simulink model "Simple_Model_Packaging_4_1"  (R2022b)
settings: Solver=VariableStepAuto  StartTime=0.0  StopTime=0.03  RelTol=1e-3
InitFcn:
  | Parameter_Initialize_4
undefined symbols (not defined in the file or in its folder): gcbh, model, rcfiltgaincompat, rsgenpoly
libraries: dspobslib x11, commdigbbndpm3 x6, commdigbbndam3 x6, simulink x5, commblkintrlv2 x4, commfilt2 x4, commsynccomp2 x3, commblkcod2 x2, commrandsrc3 x2, commseqgen3 x2, commchan3 x1, dspsigops x1
(part 1 of 2)
settings Model: Creator=89778  LastModifiedBy=z0y

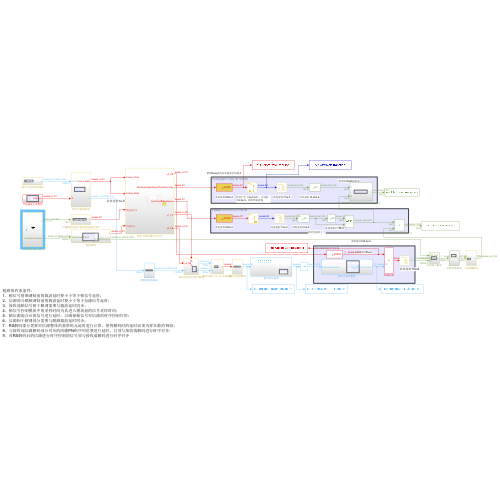
[thumbnail: Simulink's stored preview of the top-level diagram]
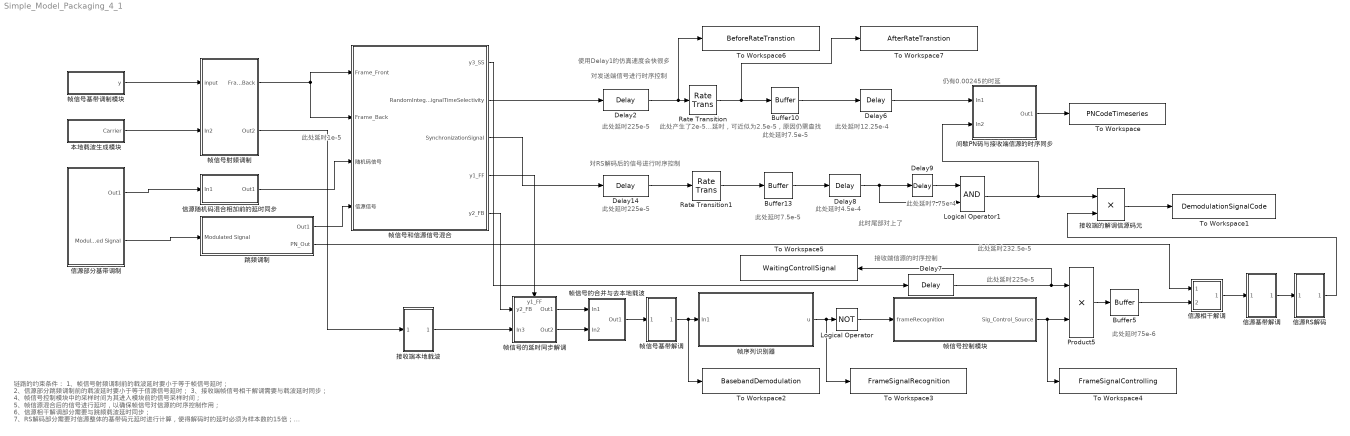
== system Simple_Model_Packaging_4_1 ==
  note: 此时尾部对上了
  note: 此处产生了2e-5延时，可近似为2.5e-5，原因仍需查找
  note: 仍有0.00245的时延
  note: 使用Delay1的仿真速度会快很多
  note: 对发送端信号进行时序控制
  note: 链路的约束条件：
      | 1、帧信号射频调制前的载波延时要小于等于帧信号延时；
      | 2、信源部分跳频调制前的载波延时要小于等于信源信号延时；
      | 3、接收端帧信号相干解调需要与载波延时同步；
      | 4、帧信号控制模块中的采样时间为其进入模块前的信号采样时间；
      | 5、帧信源混合后的信号进行延时，以确保帧信号对信源的时序控制作用；
      | 6、信源相干解调部分需要与跳频载波延时同步；
      | 7、RS解码部分需要对信源整体的基带码元延时进行计算，使得解码时的延时必须为样本数的15倍；
      | 8、与接收端信源解码部分对应的间歇PN码序列也要进行延时，且须与接收端解码进行时序对齐；
      | 9、对RS解码后的信源进行时序控制的信号须与接收端解码进行时序对齐
  note: 此处延时75e-6
  note: 此处延时1e-5
  note: 对RS解码后的信号进行时序控制
  note: 接收端信源的时序控制
  note: 此处延时225e-5
  note: 此处延时225e-5
  note: 此处延时7.5e-5
  note: 此处延时7.5e-5
  note: 此处延时7.75e-4
  note: 此处延时232.5e-5
  note: 此处延时225e-5
  note: 此处延时12.25e-4
  note: 此处延时4.5e-4
  Buffer10 : Buffer  N=model.parameter.Buffer10.Output_buffer_size  OutputFrames=off
  Buffer13 : Buffer  N=model.parameter.Buffer13.Output_buffer_size  OutputFrames=off
  Buffer5 : Buffer  N=model.parameter.Beffer5.Output_buffer_size  OutputFrames=off
  Delay14 : dspobslib/Delay  InputProcessing=Columns as channels (frame based)  dly_unit=Samples  delay=model.parameter.Delay14.Output_buffer_size  ic_detail=off  dif_ic_for_ch=on  dif_ic_for_dly=off  ic=0  reset_popup=None
  Delay2 : dspobslib/Delay  InputProcessing=Columns as channels (frame based)  dly_unit=Samples  delay=model.parameter.Delay2.Output_buffer_size  ic_detail=off  dif_ic_for_ch=on  dif_ic_for_dly=off  ic=0  reset_popup=None
  Delay6 : dspobslib/Delay  InputProcessing=Columns as channels (frame based)  dly_unit=Samples  delay=model.parameter.Delay6.Output_buffer_size  ic_detail=off  dif_ic_for_ch=on  dif_ic_for_dly=off  ic=0  reset_popup=None
  Delay7 : dspobslib/Delay  InputProcessing=Columns as channels (frame based)  dly_unit=Samples  delay=model.parameter.Delay7.samples_length  ic_detail=off  dif_ic_for_ch=on  dif_ic_for_dly=off  ic=0  reset_popup=None
  Delay8 : dspobslib/Delay  InputProcessing=Columns as channels (frame based)  dly_unit=Samples  delay=model.parameter.Delay8.Output_buffer_size  ic_detail=off  dif_ic_for_ch=on  dif_ic_for_dly=off  ic=0  reset_popup=None
  Delay9 : dspobslib/Delay  InputProcessing=Columns as channels (frame based)  dly_unit=Samples  delay=model.parameter.Delay9.Output_buffer_size  ic_detail=off  dif_ic_for_ch=on  dif_ic_for_dly=off  ic=0  reset_popup=None
  Logical Operator : Logic  Operator=NOT  AllPortsSameDT=off  OutDataTypeStr=boolean
  Logical Operator1 : Logic  AllPortsSameDT=off  OutDataTypeStr=boolean
  Product5 : Product
  Rate Transition : RateTransition  OutPortSampleTime=model.parameter.Rate_Transition.Ts
  Rate Transition1 : RateTransition  OutPortSampleTime=model.parameter.Rate_Transition1.Ts
  To Workspace : ToWorkspace  VariableName=PNCodeTimeseries  SaveFormat=Timeseries  SampleTime=-1
  To Workspace1 : ToWorkspace  VariableName=DemodulationSignalCode  SaveFormat=Timeseries  SampleTime=-1
  To Workspace2 : ToWorkspace  VariableName=BasebandDemodulation  SaveFormat=Timeseries  SampleTime=-1
  To Workspace3 : ToWorkspace  VariableName=FrameSignalRecognition  SaveFormat=Timeseries  SampleTime=-1
  To Workspace4 : ToWorkspace  VariableName=FrameSignalControlling  SaveFormat=Timeseries  SampleTime=-1
  To Workspace5 : ToWorkspace  VariableName=WaitingControllSignal  SaveFormat=Timeseries  SampleTime=-1
  To Workspace6 : ToWorkspace  VariableName=BeforeRateTranstion  SaveFormat=Timeseries  SampleTime=-1
  To Workspace7 : ToWorkspace  VariableName=AfterRateTranstion  SaveFormat=Timeseries  SampleTime=-1
  信源RS解码 : Subsystem
  信源基带解调 : Subsystem
  信源相干解调 : Subsystem
  信源部分基带调制 : Subsystem
  信源随机码混合相加前的延时同步 : Subsystem
  帧信号和信源信号混合 : Subsystem
  帧信号基带解调 : Subsystem
  帧信号基带调制模块 : Subsystem
  帧信号射频调制 : Subsystem
  帧信号控制模块 : Subsystem
  帧信号的合并与去本地载波 : Subsystem
  帧信号的延时同步解调 : Subsystem
      settings: PortSchema="{\"entries\":[{\"content\":{\"sides\":[{\"content\":{\"connectorIds\":[\"In1\",\"In2\"]},\"type\":\"ConnectorPlacement.EquallySpacedRectSide\",\"uuid\":\"7f942f1a-e4af-4868-9b8e-272828cafa58\"},{\"content\":{\"connectorIds\":[\"Out1\",\"Out2\"],\"side\":\"RIGHT\"},\"type\":\"ConnectorPlacement.EquallySpacedRectSide\",\"uuid\":\"5681018a-c54d-4fc6-9bb9-b0c232ec8fca\"},{\"content\":{\"connectorIds\":[\"In3\"],\"side\":\"TOP\"},\"type\":\"ConnectorPlacement.EquallySpacedRectSide\",\"uuid\":\"54722782-433f-4e80-acce-11fefe357297\"}]},\"type\":\"ConnectorPlacement.EquallySpacedConnector\",\"uuid\":\"571cebd7-6074-490f-8ff4-11297431766f\"}],\"packageUris\":[\"http://schema.mathworks.com/mf0/Connector/R2020b\"],\"version\":\"1.0\"}"
  帧序列识别器 : Subsystem
  接收端本地载波 : Subsystem
  接收端的解调信源码元 : Product
  本地载波生成模块 : Subsystem
  跳频调制 : Subsystem
  间歇PN码与接收端信源的时序同步 : Subsystem
  wires:
  Product5/1 -> Buffer5/1
  帧信号和信源信号混合/1(y3_SS) -> Delay7/1
  帧序列识别器/1(u) -> To Workspace3/1, Logical Operator/1
  Delay7/1 -> To Workspace5/1, Product5/1
  Buffer13/1 -> Delay8/1
  帧信号基带调制模块/1(y) -> 帧信号射频调制/1(input)
  本地载波生成模块/1(Carrier) -> 帧信号射频调制/2(In2)
  跳频调制/1(Out1) -> 帧信号和信源信号混合/4(信源信号)
  帧信号射频调制/2(Out2) -> 接收端本地载波/1(In1)
  信源部分基带调制/1(Out1) -> 信源随机码混合相加前的延时同步/1(In1)
  信源随机码混合相加前的延时同步/1(Out1) -> 帧信号和信源信号混合/3(随机码信号)
  接收端本地载波/1(Out1) -> 帧信号的延时同步解调/2(In3)
  帧信号的延时同步解调/1(Out1) -> 帧信号的合并与去本地载波/1(In1)
  帧信号的延时同步解调/2(Out2) -> 帧信号的合并与去本地载波/2(In2)
  帧信号的合并与去本地载波/1(Out1) -> 帧信号基带解调/1(In1)
  帧信号基带解调/1(Out1) -> To Workspace2/1, 帧序列识别器/1(In1)
  Logical Operator/1 -> 帧信号控制模块/1(frameRecognition)
  帧信号控制模块/1(Sig_Control_Source) -> To Workspace4/1, Product5/2
  信源RS解码/1(Out1) -> 接收端的解调信源码元/2
  Buffer5/1 -> 信源相干解调/2(In2)
  信源相干解调/1(Out1) -> 信源基带解调/1(In1)
  帧信号和信源信号混合/4(y1_FF) -> 帧信号的延时同步解调/3(y1_FF)
  帧信号和信源信号混合/5(y2_FB) -> 帧信号的延时同步解调/1(y2_FB)
  跳频调制/2(PN_Out) -> 信源相干解调/1(PN_Out)
  Delay14/1 -> Rate Transition1/1
  帧信号和信源信号混合/2(RandomIntegerSignalTimeSelectivity) -> Delay2/1
  Rate Transition/1 -> To Workspace7/1, Buffer10/1
  Delay2/1 -> To Workspace6/1, Rate Transition/1
  Rate Transition1/1 -> Buffer13/1
  帧信号和信源信号混合/3(SynchronizationSignal) -> Delay14/1
  信源基带解调/1(Out1) -> 信源RS解码/1(In1)
  Buffer10/1 -> Delay6/1
  Delay6/1 -> 间歇PN码与接收端信源的时序同步/1(In1)
  Delay9/1 -> Logical Operator1/1
  Delay8/1 -> Logical Operator1/2, Delay9/1
  信源部分基带调制/2(Modulated Signal) -> 跳频调制/1(Modulated Signal)
  帧信号射频调制/1(Frame_Back) -> 帧信号和信源信号混合/2(Frame_Back), 帧信号和信源信号混合/1(Frame_Front)
  Logical Operator1/1 -> 间歇PN码与接收端信源的时序同步/2(In2), 接收端的解调信源码元/1
  间歇PN码与接收端信源的时序同步/1(Out1) -> To Workspace/1
  接收端的解调信源码元/1 -> To Workspace1/1

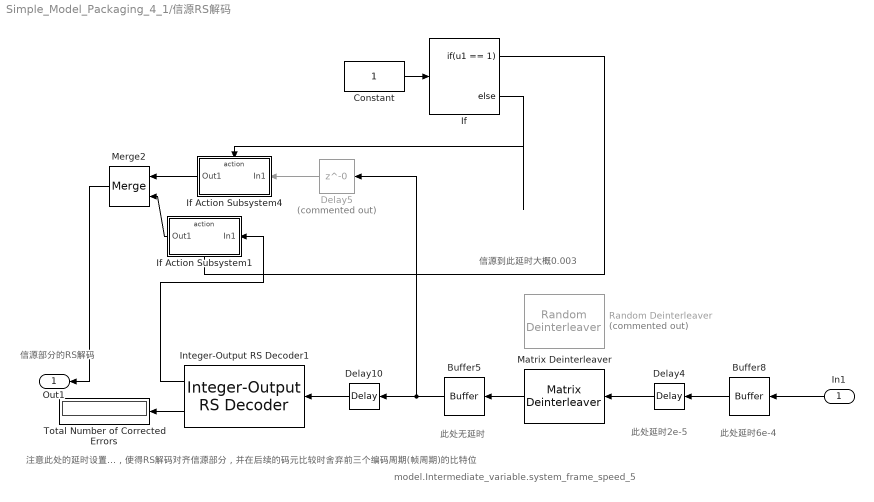
== system Simple_Model_Packaging_4_1/信源RS解码 ==
  note: 信源到此延时大概0.003
  note: model.Intermediate_variable.system_frame_speed_5
  note: 信源部分的RS解码
  note: 注意此处的延时设置，使得RS解码对齐信源部分，并在后续的码元比较时舍弃前三个编码周期(帧周期)的比特位
  note: 此处延时2e-5
  note: 此处无延时
  note: 此处延时6e-4
  In1 : Inport
  Buffer5 : Buffer  N=model.parameter.Buffer5.Output_buffer_size  OutputFrames=off
  Buffer8 : Buffer  N=model.parameter.Buffer8.Output_buffer_size  OutputFrames=off
  Constant : Constant
  Delay10 : dspobslib/Delay  InputProcessing=Columns as channels (frame based)  dly_unit=Samples  delay=model.parameter.Delay10.samples_length  ic_detail=off  dif_ic_for_ch=on  dif_ic_for_dly=off  ic=0  reset_popup=None
  Delay4 : dspobslib/Delay  InputProcessing=Columns as channels (frame based)  dly_unit=Samples  delay=model.parameter.Delay4.samples_length  ic_detail=off  dif_ic_for_ch=on  dif_ic_for_dly=off  ic=0  reset_popup=None
  Delay5 : Delay  Commented=on  DelayLength=0  InitialCondition=0  InputProcessing=Columns as channels (frame based)
  If : If  IfExpression=u1 == 1
  If Action Subsystem1 : Subsystem  TreatAsAtomicUnit=on
  If Action Subsystem4 : Subsystem  TreatAsAtomicUnit=on
  Integer-Output RS Decoder1 : commblkcod2/Integer-Output RS Decoder  n=model.parameter.Integer_Output_RS_Decoder1.Codeword_length  k=model.parameter.Integer_Output_RS_Decoder1.Message_length  specShortening=off  shortenedK=3  specGenPoly=off  genPoly=rsgenpoly(7, 3, [], [], 'double')  specPrimPoly=off  prPoly='X^3 + X + 1'  specPuncture=off  punctVec=[ones(2,1); zeros(2,1)]  specErasurePort=off  showNumErr=on
  Matrix Deinterleaver : commblkintrlv2/Matrix Deinterleaver  StatePerturbationForJacobian=1.0e-05  Nrows=model.parameter.Matrix_Deinterleaver.row_nums  Ncols=model.parameter.Matrix_Deinterleaver.col_nums
  Merge2 : Merge
  Random Deinterleaver : commblkintrlv2/Random Deinterleaver  Commented=on  StatePerturbationForJacobian=1.0e-05  N=120  seed=12345
  Total Number of Corrected Errors : Display
  Out1 : Outport
  wires:
  Integer-Output RS Decoder1/2 -> Total Number of Corrected Errors/1
  Matrix Deinterleaver/1 -> Buffer5/1
  In1/1 -> Buffer8/1
  Buffer8/1 -> Delay4/1
  Delay4/1 -> Matrix Deinterleaver/1
  Delay10/1 -> Integer-Output RS Decoder1/1
  If Action Subsystem4/1(Out1) -> Merge2/1
  Integer-Output RS Decoder1/1 -> If Action Subsystem1/1(In1)
  Buffer5/1 -> Delay5/1, Delay10/1
  Merge2/1 -> Out1/1
  Delay5/1 -> If Action Subsystem4/1(In1)
  If Action Subsystem1/1(Out1) -> Merge2/2
  If/1 -> If Action Subsystem1/Action
  Constant/1 -> If/1
  If/2 -> If Action Subsystem4/Action

== system Simple_Model_Packaging_4_1/信源基带解调 ==
  note: 接收端信源的基带解调
  note: 此处延时2.5e-5
  In1 : Inport
  Baseband Signal Selector Rx : Subsystem
  Merge : Merge  Inputs=3
  OQPSK Demodulator Baseband : commdigbbndpm3/OQPSK Demodulator Baseband  Commented=on  OutType=Integer  Ph=0  Mapping=Gray  pulseShape=Half sine  num=[0.7071, 0.7071]  rolloff=0.2  filterSpan=10  sps=2  RateOptions=Enforce single-rate processing  outDtype2=double
  QPSK Demodulator Baseband : commdigbbndpm3/QPSK Demodulator Baseband  Commented=on  OutType=Integer  DecType=Hard decision  VarSource=Dialog  Variance=1  Dec=Gray  Ph=pi/4  outDtype1=Inherit via internal rule  outDtype2=Inherit via internal rule  derotateFactorWordLen=16  derotateFactorDataTypeStr=Inherit: Same word length as input  derotateFactorLastDataTypeStr=Inherit: Same word length as input
  Raised Cosine Receive Filter1 : commfilt2/Raised Cosine Receive Filter  filtType=Square root  R=model.parameter.Raised_Cosine_Receive_Filter1.Rolloff_factor  filtSpan=model.parameter.Raised_Cosine_Receive_Filter1.Filter_span_in_symbols  N=model.parameter.Raised_Cosine_Receive_Filter1.Input_samples_per_symbol  downFactor=model.parameter.Raised_Cosine_Receive_Filter1.Decimation_fatocr  downOffset=0  filterGain=rcfiltgaincompat(gcbh)  InputProcessing=Columns as channels (frame based)  RateOptions=Enforce single-rate processing  framing=Mute  checkCoeff=off  variableName=rcRxFilt1  currentFiltSpan=10  D=5  inputOffset=0  sampMode=Mute  saveAsFlag=0  rateMode=Downsampling  checkGain=Normalized  launchFVT=on  roundingMode=Floor  overflowMode=off  coeffDataTypeStr=Inherit: Same word length as input  coeffMin=[]  coeffMax=[]  coeffLastDataTypeStr=Inherit: Same word length as input  accumDataTypeStr=Inherit: Same as product output  accumLastDataTypeStr=Inherit: Same as product output  outputDataTypeStr=Inherit: Same as accumulator  outputMin=[]  outputMax=[]  outputLastDataTypeStr=Inherit: Same as accumulator
  Out1 : Outport
  wires:
  Merge/1 -> Out1/1
  In1/1 -> Raised Cosine Receive Filter1/1
  Raised Cosine Receive Filter1/1 -> OQPSK Demodulator Baseband/1, QPSK Demodulator Baseband/1, Baseband Signal Selector Rx/1(In1)
  OQPSK Demodulator Baseband/1 -> Merge/3
  Baseband Signal Selector Rx/1(Out1) -> Merge/1
  QPSK Demodulator Baseband/1 -> Merge/2

== system Simple_Model_Packaging_4_1/信源相干解调 ==
  note: 接收端信源的相干解调
  PN_Out : Inport
  In2 : Inport  Port=2
  Conj1 : Math  Operator=conj
  Delay3 : dspobslib/Delay  InputProcessing=Columns as channels (frame based)  dly_unit=Samples  delay=model.parameter.Delay3.samples_length  ic_detail=off  dif_ic_for_ch=on  dif_ic_for_dly=off  ic=0  reset_popup=None
  Product3 : Product
  Out1 : Outport
  wires:
  PN_Out/1 -> Delay3/1
  Conj1/1 -> Product3/1
  In2/1 -> Product3/2
  Product3/1 -> Out1/1
  Delay3/1 -> Conj1/1

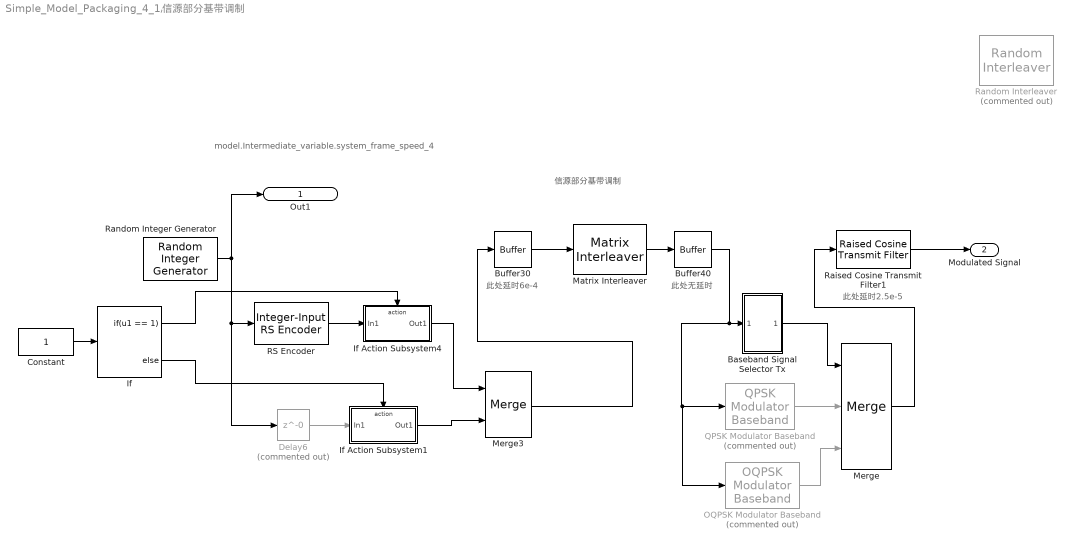
== system Simple_Model_Packaging_4_1/信源部分基带调制 ==
  note: model.Intermediate_variable.system_frame_speed_4
  note: 信源部分基带调制
  note: 此处延时2.5e-5
  note: 此处延时6e-4
  note: 此处无延时
  Baseband Signal Selector Tx : Subsystem
  Buffer30 : Buffer  N=model.parameter.Buffer30.Output_buffer_size  OutputFrames=off
  Buffer40 : Buffer  N=model.parameter.Buffer40.Output_buffer_size  OutputFrames=off
  Constant : Constant
  Delay6 : Delay  Commented=on  DelayLength=0  InitialCondition=0
  If : If  IfExpression=u1 == 1
  If Action Subsystem1 : Subsystem  TreatAsAtomicUnit=on
  If Action Subsystem4 : Subsystem  TreatAsAtomicUnit=on
  Matrix Interleaver : commblkintrlv2/Matrix Interleaver  StatePerturbationForJacobian=1.0e-05  Nrows=model.parameter.Matrix_Interleaver.row_nums  Ncols=model.parameter.Matrix_Interleaver.col_nums
  Merge : Merge  Inputs=3
  Merge3 : Merge
  OQPSK Modulator Baseband : commdigbbndpm3/OQPSK Modulator Baseband  Commented=on  InType=Integer  Ph=0  Mapping=Gray  pulseShape=Half sine  num=[0.7071, 0.7071]  rolloff=0.2  filterSpan=10  sps=2  RateOptions=Enforce single-rate processing  outDtype=double
  QPSK Modulator Baseband : commdigbbndpm3/QPSK Modulator Baseband  Commented=on  InType=Integer  Enc=Gray  Ph=pi/4  outDtype=double  outWordLen=16  outUDDataType=sfix(16)  outFracLenMode=Best precision  outFracLen=15  outDataTypeStr=double  outLastDataTypeStr=double
  RS Encoder : commblkcod2/Integer-Input RS Encoder  n=model.parameter.RS_Encoder.Codeword_length  k=model.parameter.RS_Encoder.Message_length  specShortening=off  shortenedK=3  specGenPoly=off  genPoly=rsgenpoly(7,3)  specPrimPoly=off  prPoly=[1 0 1 1]  specPuncture=off  punctVec=[ones(2,1); zeros(2,1)]
  Raised Cosine Transmit Filter1 : commfilt2/Raised Cosine Transmit Filter  filtType=Square root  R=model.parameter.Raised_Cosine_Transmit_Filter1.Rolloff_factor  filtSpan=model.parameter.Raised_Cosine_Transmit_Filter1.Filter_span_in_symbols  N=model.parameter.Raised_Cosine_Transmit_Filter1.Input_samples_per_symbol  filterGain=rcfiltgaincompat(gcbh)  InputProcessing=Columns as channels (frame based)  RateOptions=Enforce single-rate processing  framing=Mute  checkCoeff=off  variableName=rcTxFilt1  checkGain=Normalized  sampMode=Mute  saveAsFlag=0  currentFiltSpan=10  D=(10)/2  launchFVT=on  roundingMode=Floor  overflowMode=off  coeffDataTypeStr=Inherit: Same word length as input  coeffMin=[]  coeffMax=[]  coeffLastDataTypeStr=Inherit: Same word length as input  outputDataTypeStr=Inherit: Same as accumulator  outputMin=[]  outputMax=[]  outputLastDataTypeStr=Inherit: Same as accumulator
  Random Interleaver : commblkintrlv2/Random Interleaver  Commented=on  StatePerturbationForJacobian=1.0e-05  N=120  seed=12345
  Random Integer Generator : commrandsrc3/Random Integer Generator  SetSize=model.parameter.Random_Integer_Generator.Set_size  SeedSource=Auto  Seed=4  SampleTime=model.parameter.Random_Integer_Generator.SignalSourceTs  SamplesPerFrame=model.parameter.Random_Integer_Generator.Samples_per_frame  OutputDataType=double  SimulateUsing=Interpreted execution
  Out1 : Outport
  Modulated Signal : Outport  Port=2
  wires:
  Raised Cosine Transmit Filter1/1 -> Modulated Signal/1
  Merge3/1 -> Buffer30/1
  Buffer30/1 -> Matrix Interleaver/1
  Matrix Interleaver/1 -> Buffer40/1
  Random Integer Generator/1 -> RS Encoder/1, Delay6/1, Out1/1
  Baseband Signal Selector Tx/1(Out1) -> Merge/1
  OQPSK Modulator Baseband/1 -> Merge/3
  QPSK Modulator Baseband/1 -> Merge/2
  Buffer40/1 -> Baseband Signal Selector Tx/1(In1), OQPSK Modulator Baseband/1, QPSK Modulator Baseband/1
  Merge/1 -> Raised Cosine Transmit Filter1/1
  If Action Subsystem4/1(Out1) -> Merge3/1
  RS Encoder/1 -> If Action Subsystem4/1(In1)
  Delay6/1 -> If Action Subsystem1/1(In1)
  If Action Subsystem1/1(Out1) -> Merge3/2
  Constant/1 -> If/1
  If/2 -> If Action Subsystem1/Action
  If/1 -> If Action Subsystem4/Action

== system Simple_Model_Packaging_4_1/信源随机码混合相加前的延时同步 ==
  note: 此处延时2.5e-5
  note: 该条支路对发送端的随机码序列进行同步时域处理，用于判断链路
      | 的误码率
  note: 此处无延时
  In1 : Inport
  Buffer14 : Buffer  N=model.parameter.Buffer14.Output_buffer_size  OutputFrames=off
  Delay11 : dspobslib/Delay  InputProcessing=Columns as channels (frame based)  dly_unit=Samples  delay=model.parameter.Delay11.samples_length  ic_detail=off  dif_ic_for_ch=on  dif_ic_for_dly=off  ic=0  reset_popup=None
  Rate Transition2 : RateTransition  OutPortSampleTime=model.Intermediate_variable.system_frame_speed_3
  Out1 : Outport
  wires:
  In1/1 -> Delay11/1
  Buffer14/1 -> Rate Transition2/1
  Rate Transition2/1 -> Out1/1
  Delay11/1 -> Buffer14/1

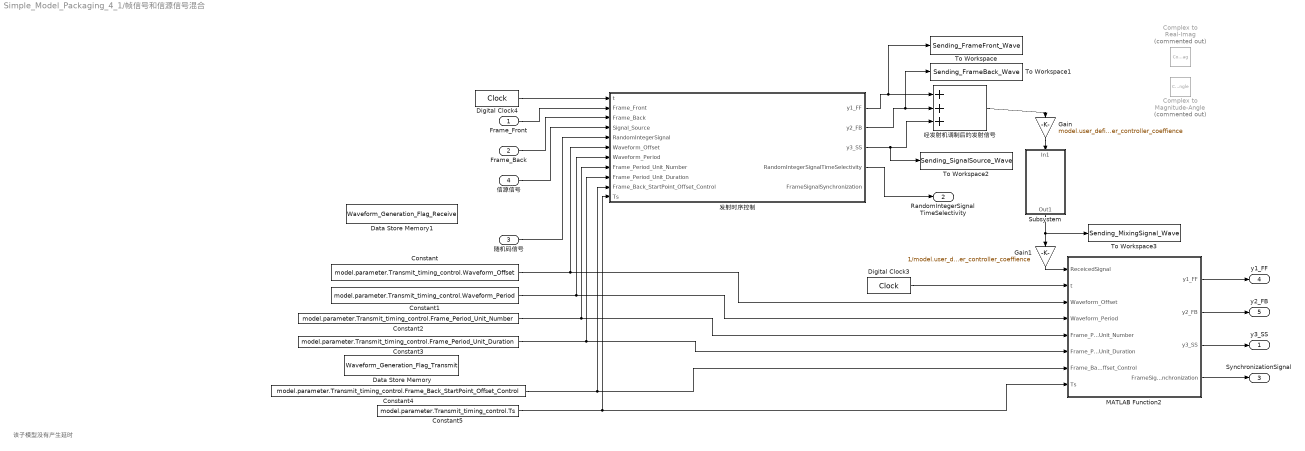
== system Simple_Model_Packaging_4_1/帧信号和信源信号混合 ==
  note: 该子模型没有产生延时
  Frame_Front : Inport
  Frame_Back : Inport  Port=2
  随机码信号 : Inport  Port=3
  信源信号 : Inport  Port=4
  Complex to Magnitude-Angle : ComplexToMagnitudeAngle  Commented=on
  Complex to Real-Imag : ComplexToRealImag  Commented=on
  Constant : Constant  Value=model.parameter.Transmit_timing_control.Waveform_Offset
  Constant1 : Constant  Value=model.parameter.Transmit_timing_control.Waveform_Period
  Constant2 : Constant  Value=model.parameter.Transmit_timing_control.Frame_Period_Unit_Number
  Constant3 : Constant  Value=model.parameter.Transmit_timing_control.Frame_Period_Unit_Duration
  Constant4 : Constant  Value=model.parameter.Transmit_timing_control.Frame_Back_StartPoint_Offset_Control
  Constant5 : Constant  Value=model.parameter.Transmit_timing_control.Ts
  Data Store Memory : DataStoreMemory  DataStoreName=Waveform_Generation_Flag_Transmit  WriteAfterWriteMsg=warning  ShowAdditionalParam=off  OutDataTypeStr=int8
  Data Store Memory1 : DataStoreMemory  DataStoreName=Waveform_Generation_Flag_Receive  WriteAfterWriteMsg=warning  ShowAdditionalParam=off  OutDataTypeStr=int8
  Digital Clock3 : DigitalClock  SampleTime=model.parameter.Digital_Clock4.Ts
  Digital Clock4 : DigitalClock  SampleTime=model.parameter.Digital_Clock4.Ts
  Gain : Gain  Gain=model.user_defined.TR.Sig_power_controller_coeffience
  Gain1 : Gain  Gain=1/model.user_defined.TR.Sig_power_controller_coeffience
  MATLAB Function2 : MATLAB Function  TreatAsAtomicUnit=on
  Subsystem : Subsystem
  To Workspace : ToWorkspace  VariableName=Sending_FrameFront_Wave  SaveFormat=Timeseries  SampleTime=-1
  To Workspace1 : ToWorkspace  VariableName=Sending_FrameBack_Wave  SaveFormat=Timeseries  SampleTime=-1
  To Workspace2 : ToWorkspace  VariableName=Sending_SignalSource_Wave  SaveFormat=Timeseries  SampleTime=-1
  To Workspace3 : ToWorkspace  VariableName=Sending_MixingSignal_Wave  SaveFormat=Timeseries  SampleTime=-1
  发射时序控制 : MATLAB Function  TreatAsAtomicUnit=on
  经发射机调制后的发射信号 : Sum  Inputs=+++
  y3_SS : Outport
  RandomIntegerSignalTimeSelectivity : Outport  Port=2
  SynchronizationSignal : Outport  Port=3
  y1_FF : Outport  Port=4
  y2_FB : Outport  Port=5
  wires:
  Constant5/1 -> 发射时序控制/11(Ts), MATLAB Function2/8(Ts)
  Constant2/1 -> MATLAB Function2/5(Frame_Period_Unit_Number), 发射时序控制/8(Frame_Period_Unit_Number)
  Digital Clock4/1 -> 发射时序控制/1(t)
  Constant/1 -> MATLAB Function2/3(Waveform_Offset), 发射时序控制/6(Waveform_Offset)
  Frame_Front/1 -> 发射时序控制/2(Frame_Front)
  Frame_Back/1 -> 发射时序控制/3(Frame_Back)
  信源信号/1 -> 发射时序控制/4(Signal_Source)
  随机码信号/1 -> 发射时序控制/5(RandomIntegerSignal)
  Constant1/1 -> MATLAB Function2/4(Waveform_Period), 发射时序控制/7(Waveform_Period)
  Constant3/1 -> MATLAB Function2/6(Frame_Period_Unit_Duration), 发射时序控制/9(Frame_Period_Unit_Duration)
  Constant4/1 -> MATLAB Function2/7(Frame_Back_StartPoint_Offset_Control), 发射时序控制/10(Frame_Back_StartPoint_Offset_Control)
  发射时序控制/1(y1_FF) -> 经发射机调制后的发射信号/1, To Workspace/1
  发射时序控制/2(y2_FB) -> To Workspace1/1, 经发射机调制后的发射信号/2
  Digital Clock3/1 -> MATLAB Function2/2(t)
  发射时序控制/3(y3_SS) -> To Workspace2/1, 经发射机调制后的发射信号/3
  发射时序控制/4(RandomIntegerSignalTimeSelectivity) -> RandomIntegerSignalTimeSelectivity/1
  MATLAB Function2/1(y1_FF) -> y1_FF/1
  MATLAB Function2/2(y2_FB) -> y2_FB/1
  MATLAB Function2/3(y3_SS) -> y3_SS/1
  MATLAB Function2/4(FrameSignalSynchronization) -> SynchronizationSignal/1
  经发射机调制后的发射信号/1 -> Gain/1
  Subsystem/1(Out1) -> To Workspace3/1, Gain1/1
  Gain/1 -> Subsystem/1(In1)
  Gain1/1 -> MATLAB Function2/1(ReceicedSignal)

== system Simple_Model_Packaging_4_1/帧信号基带解调 ==
  note: 此处延时为20e-4
  note: 帧信号的基带解调
  note: 此处延时为2.5e-4
  note: 此处无延时
  In1 : Inport
  Buffer1 : Buffer  N=model.parameter.Buffer11.Output_buffer_size  OutputFrames=off
  Buffer7 : Buffer  N=model.parameter.Buffer7.Output_buffer_size  OutputFrames=off
  M-PAM Demodulator Baseband : commdigbbndam3/M-PAM Demodulator Baseband  M=model.parameter.M_PAM_Demodulator_Baseband.M_ary_number  OutType=Integer  Dec=Gray  PowType=Min. distance between symbols  MinDist=model.parameter.M_PAM_Demodulator_Baseband.Minimum_distance  AvgPow=1  PeakPow=1  outDtype1=Inherit via internal rule  outDtype2=Inherit via internal rule  denormFactorWordLen=16  denormFactorDataTypeStr=Inherit: Same word length as input  denormFactorLastDataTypeStr=Inherit: Same word length as input  prodOutWordLen=16  prodOutRoundingMode=Floor  prodOutOverflowMode=Wrap  prodOutOvFlMode=off  prodOutOvFlModeLastStrValue=off  sumWordLen=16
  MATLAB Function3 : MATLAB Function  TreatAsAtomicUnit=on
  Raised Cosine Receive Filter : commfilt2/Raised Cosine Receive Filter  filtType=Square root  R=model.parameter.Raised_Cosine_Receive_Filter.Rolloff_factor  filtSpan=model.parameter.Raised_Cosine_Receive_Filter.Filter_span_in_symbols  N=model.parameter.Raised_Cosine_Receive_Filter.Input_samples_per_symbol  downFactor=model.parameter.Raised_Cosine_Receive_Filter.Decimation_factor  downOffset=0  filterGain=rcfiltgaincompat(gcbh)  InputProcessing=Columns as channels (frame based)  RateOptions=Enforce single-rate processing  framing=Mute  checkCoeff=off  variableName=rcRxFilt  currentFiltSpan=10  D=5  inputOffset=0  sampMode=Mute  saveAsFlag=0  rateMode=Downsampling  checkGain=Normalized  launchFVT=on  roundingMode=Floor  overflowMode=off  coeffDataTypeStr=Inherit: Same word length as input  coeffMin=[]  coeffMax=[]  coeffLastDataTypeStr=Inherit: Same word length as input  accumDataTypeStr=Inherit: Same as product output  accumLastDataTypeStr=Inherit: Same as product output  outputDataTypeStr=Inherit: Same as accumulator  outputMin=[]  outputMax=[]  outputLastDataTypeStr=Inherit: Same as accumulator
  Out1 : Outport
  wires:
  Raised Cosine Receive Filter/1 -> M-PAM Demodulator Baseband/1
  In1/1 -> Buffer7/1
  M-PAM Demodulator Baseband/1 -> Out1/1
  Buffer7/1 -> MATLAB Function3/1(input)
  MATLAB Function3/1(y) -> Buffer1/1
  Buffer1/1 -> Raised Cosine Receive Filter/1

== system Simple_Model_Packaging_4_1/帧信号基带调制模块 ==
  note: model.Intermediate_variable.system_frame_speed_2
  note: model.Intermediate_variable.system_frame_speed_1
  note: 此处buffer的设计需要让插值后buffer的速率等于帧信号的编码速率
  note: 此处产生了200e-5的延时
  note: 帧信号基带调制模块
  note: 此处产生了2.5e-4延时
  note: 此处无延时
  Buffer1 : Buffer  N=model.parameter.Buffer1.Output_buffer_size  OutputFrames=off
  Buffer12 : Buffer  N=model.parameter.Buffer12.Output_buffer_size  OutputFrames=off
  M-PAM Modulator Baseband : commdigbbndam3/M-PAM Modulator Baseband  M=model.parameter.M_PAM_Modulator_Baseband.M_ary_number  InType=Integer  Enc=Gray  PowType=Min. distance between symbols  MinDist=model.parameter.M_PAM_Modulator_Baseband.Minimum_distance  AvgPow=1  PeakPow=1  outDtype=double  outWordLen=16  outUDDataType=sfix(16)  outFracLenMode=Best precision  outFracLen=15  outDataTypeStr=double  outLastDataTypeStr=double
  Raised Cosine Transmit Filter : commfilt2/Raised Cosine Transmit Filter  filtType=Square root  R=model.parameter.Raised_Cosine_Transmit_Filter.Rolloff_factor  filtSpan=model.parameter.Raised_Cosine_Transmit_Filter.Filter_span_in_symbols  N=model.parameter.Raised_Cosine_Transmit_Filter.Output_samples_per_symbol  filterGain=rcfiltgaincompat(gcbh)  InputProcessing=Columns as channels (frame based)  RateOptions=Enforce single-rate processing  framing=Mute  checkCoeff=off  variableName=rcTxFilt  checkGain=Normalized  sampMode=Mute  saveAsFlag=0  currentFiltSpan=10  D=(10)/2  launchFVT=on  roundingMode=Floor  overflowMode=off  coeffDataTypeStr=Inherit: Same word length as input  coeffMin=[]  coeffMax=[]  coeffLastDataTypeStr=Inherit: Same word length as input  outputDataTypeStr=Inherit: Same as accumulator  outputMin=[]  outputMax=[]  outputLastDataTypeStr=Inherit: Same as accumulator
  rateTransitionUserDefined : MATLAB Function  TreatAsAtomicUnit=on
  帧信号编码码元 : simulink/Sources/Repeating Sequence Stair  OutValues=model.parameter.Repeating_Sequence_Stair.output_vector  tsamp=model.parameter.Repeating_Sequence_Stair.CodeTs  OutMin=[]  OutMax=[]  OutDataTypeStr=double  OutputDataTypeScalingMode=double  OutDataType=fixdt(0,8)  ConRadixGroup=Best Precision: Vector-wise  OutScaling=2^-12
  y : Outport
  wires:
  帧信号编码码元/1 -> M-PAM Modulator Baseband/1
  M-PAM Modulator Baseband/1 -> Raised Cosine Transmit Filter/1
  Raised Cosine Transmit Filter/1 -> Buffer12/1  "基带帧信号"
  rateTransitionUserDefined/1(y) -> Buffer1/1
  Buffer1/1 -> y/1
  Buffer12/1 -> rateTransitionUserDefined/1(input)

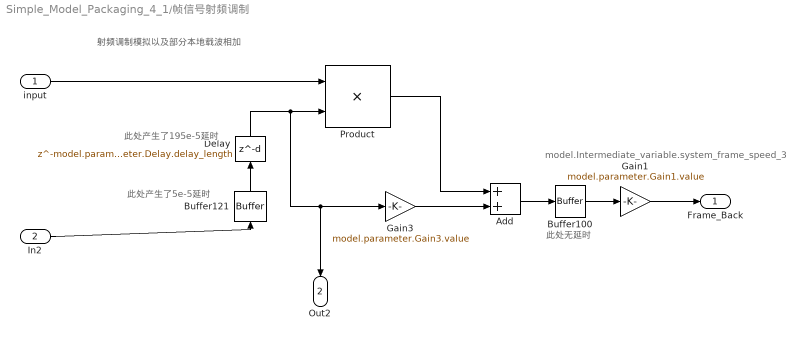
== system Simple_Model_Packaging_4_1/帧信号射频调制 ==
  note: model.Intermediate_variable.system_frame_speed_3
  note: 此处无延时
  note: 此处产生了5e-5延时
  note: 射频调制模拟以及部分本地载波相加
  note: 此处产生了195e-5延时
  input : Inport
  In2 : Inport  Port=2
  Add : Sum
  Buffer100 : Buffer  N=model.parameter.Buffer100.Output_buffer_size  OutputFrames=off
  Buffer121 : Buffer  N=model.parameter.Buffer121.Output_buffer_size  OutputFrames=off
  Delay : Delay  DelayLength=model.parameter.Delay.delay_length  InputProcessing=Columns as channels (frame based)
  Gain1 : Gain  Gain=model.parameter.Gain1.value
  Gain3 : Gain  Gain=model.parameter.Gain3.value
  Product : Product
  Frame_Back : Outport
  Out2 : Outport  Port=2
  wires:
  In2/1 -> Buffer121/1
  Product/1 -> Add/1
  Gain3/1 -> Add/2
  Buffer121/1 -> Delay/1
  Add/1 -> Buffer100/1
  Buffer100/1 -> Gain1/1
  input/1 -> Product/1
  Delay/1 -> Gain3/1, Out2/1, Product/2
  Gain1/1 -> Frame_Back/1

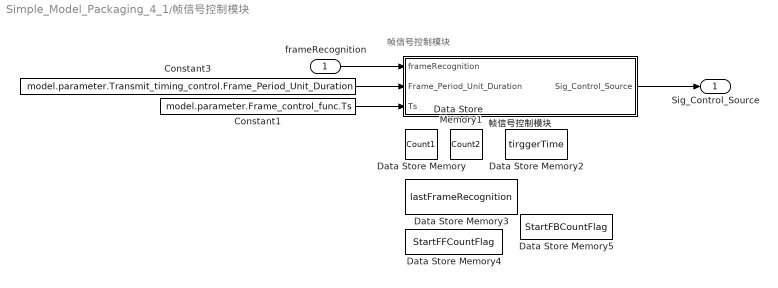
== system Simple_Model_Packaging_4_1/帧信号控制模块 ==
  note: 帧信号控制模块
  frameRecognition : Inport
  Constant1 : Constant  Value=model.parameter.Frame_control_func.Ts
  Constant3 : Constant  Value=model.parameter.Transmit_timing_control.Frame_Period_Unit_Duration
  Data Store Memory : DataStoreMemory  DataStoreName=Count1  WriteAfterWriteMsg=warning  ShowAdditionalParam=off  OutDataTypeStr=uint64
  Data Store Memory1 : DataStoreMemory  DataStoreName=Count2  WriteAfterWriteMsg=warning  ShowAdditionalParam=off  OutDataTypeStr=uint64
  Data Store Memory2 : DataStoreMemory  DataStoreName=tirggerTime  WriteAfterWriteMsg=warning  ShowAdditionalParam=off  OutDataTypeStr=int64
  Data Store Memory3 : DataStoreMemory  DataStoreName=lastFrameRecognition  WriteAfterWriteMsg=warning  ShowAdditionalParam=off  OutDataTypeStr=int8
  Data Store Memory4 : DataStoreMemory  DataStoreName=StartFFCountFlag  WriteAfterWriteMsg=warning  ShowAdditionalParam=off  OutDataTypeStr=int8
  Data Store Memory5 : DataStoreMemory  DataStoreName=StartFBCountFlag  WriteAfterWriteMsg=warning  ShowAdditionalParam=off  OutDataTypeStr=int8
  帧信号控制模块 : MATLAB Function  TreatAsAtomicUnit=on
  Sig_Control_Source : Outport
  wires:
  frameRecognition/1 -> 帧信号控制模块/1(frameRecognition)
  帧信号控制模块/1(Sig_Control_Source) -> Sig_Control_Source/1
  Constant3/1 -> 帧信号控制模块/2(Frame_Period_Unit_Duration)
  Constant1/1 -> 帧信号控制模块/3(Ts)

== system Simple_Model_Packaging_4_1/帧信号的合并与去本地载波 ==
  note: 此处无延时
  note: 接收端去本地载波
  In1 : Inport
  In2 : Inport  Port=2
  Add1 : Sum
  Add4 : Sum  Inputs=+-
  Buffer6 : Buffer  N=model.parameter.Buffer6.Output_buffer_size  OutputFrames=off
  Constant1 : Constant  Value=model.parameter.Constant1.value
  Gain2 : Gain  Gain=model.parameter.Gain2.value
  Out1 : Outport
  wires:
  In1/1 -> Add1/1
  Add4/1 -> Buffer6/1
  Buffer6/1 -> Out1/1
  Constant1/1 -> Add4/2
  Add1/1 -> Gain2/1
  In2/1 -> Add1/2
  Gain2/1 -> Add4/1

== system Simple_Model_Packaging_4_1/帧信号的延时同步解调 ==
  note: 此处延时5e-6
  note: 接收端帧头帧尾信号分别相干解调
  note: 此处延时5e-6
  note: 此处延时10e-6
  y2_FB : Inport
  In3 : Inport  Port=2
  y1_FF : Inport  Port=3
  Buffer3 : Buffer  N=model.parameter.Buffer3.Output_buffer_size  OutputFrames=off
  Buffer4 : Buffer  N=model.parameter.Buffer4.Output_buffer_size  OutputFrames=off
  Product1 : Product
  Product2 : Product
  Out1 : Outport
  Out2 : Outport  Port=2
  wires:
  In3/1 -> Product2/1, Product1/1
  Buffer3/1 -> Product1/2
  Product1/1 -> Out1/1
  Product2/1 -> Out2/1
  y2_FB/1 -> Buffer4/1
  y1_FF/1 -> Buffer3/1
  Buffer4/1 -> Product2/2

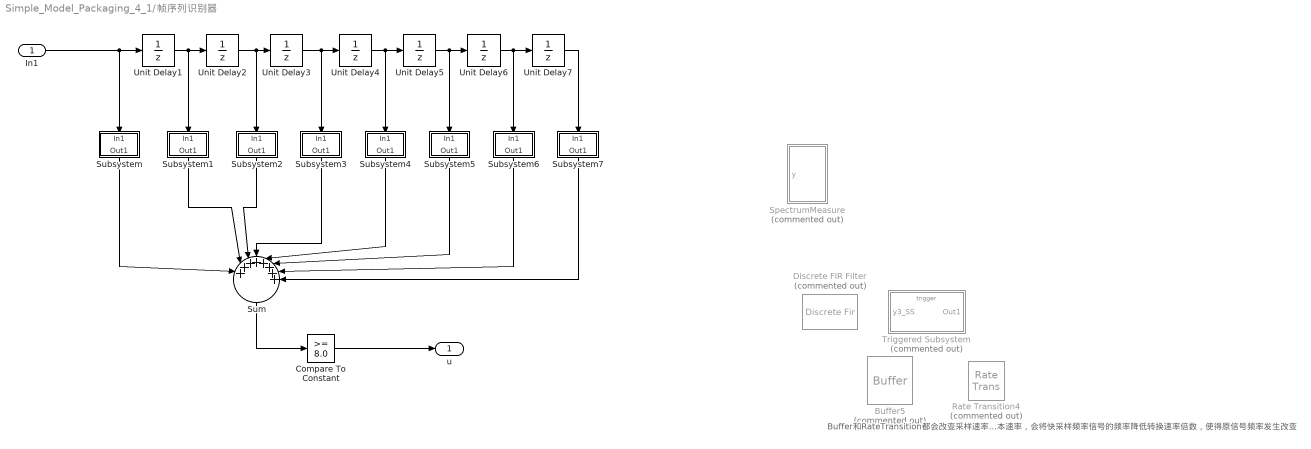
== system Simple_Model_Packaging_4_1/帧序列识别器 ==
  note: Buffer和RateTransition都会改变采样速率，但是Buffer不会改变原信号的频率，只会改变帧信号内的样本数，会额外引入延时，其改变的速率为帧速率，样本速率并没有改变，但RateTransition是直接改变样本速率，会将快采样频率信号的频率降低转换速率倍数，使得原信号频率发生改变
  In1 : Inport
  Buffer5 : Buffer  Commented=on  N=100  OutputFrames=off
  Compare To Constant : simulink/Logic and Bit Operations/Compare To Constant  relop=>=  const=8.0  OutDataTypeStr=boolean
  Discrete FIR Filter : DiscreteFir  Commented=on  Coefficients="[0\t0\t0\t0\t0\t0\t0\t0\t0\t0\t0\t0\t0\t0\t0\t0\t0\t0\t0\t0\t0\t0\t0\t0\t0\t0\t0\t0\t0\t0\t0\t0\t0\t0\t0\t0\t0\t0\t0\t0\t0\t0\t0\t0\t0\t0\t0\t0\t0\t0\t0\t0\t0\t0\t0\t0\t0\t0\t0\t0\t0\t0\t0\t0\t0\t0\t0\t0\t0\t0\t0\t0\t0\t0\t0\t0\t0\t0\t0\t0\t0\t0\t0\t0\t0\t0\t0\t0\t0\t0\t0\t0\t0\t0\t0\t0\t0\t0\t0\t0\t0\t0\t0\t0\t0\t0\t0\t0\t0\t0\t0\t6.10351562500000e-05\t6.10351562500000e-05\t6.10351562500000e-05\t6.10351562500000e-05\t6.10351562500000e-05\t6.10351562500000e-05\t6.10351562500000e-05\t6.10351562500000e-05\t6.10351562500000e-05\t6.10351562500000e-05\t6.10351562500000e-05\t6.10351562500000e-05\t6.10351562500000e-05\t6.10351562500000e-05\t0.000122070312500000\t0.000122070312500000\t0.000122070312500000\t0.000122070312500000\t0.000122070312500000\t0.000122070312500000\t0.000122070312500000\t0.000122070312500000\t0.000122070312500000\t0.000183105468750000\t0.000183105468750000\t0.000183105468750000\t0.000183105468750000\t0.000183105468750000\t0.000183105468750000\t0.000183105468750000\t0.000183105468750000\t0.000244140625000000\t0.000244140625000000\t0.000244140625000000\t0.000244140625000000\t0.000244140625000000\t0.000244140625000000\t0.000305175781250000\t0.000305175781250000\t0.000305175781250000\t0.000305175781250000\t0.000305175781250000\t0.000366210937500000\t0.000366210937500000\t0.000366210937500000\t0.000366210937500000\t0.000366210937500000\t0.000427246093750000\t0.000427246093750000\t0.000427246093750000\t0.000427246093750000\t0.000427246093750000\t0.000488281250000000\t0.000488281250000000\t0.000488281250000000\t0.000488281250000000\t0.000549316406250000\t0.000549316406250000\t0.000549316406250000\t0.000610351562500000\t0.000610351562500000\t0.000610351562500000\t0.000610351562500000\t0.000671386718750000\t0.000671386718750000\t0.000671386718750000\t0.000732421875000000\t0.000732421875000000\t0.000732421875000000\t0.000793457031250000\t0.000793457031250000\t0.000793457031250000\t0.000854492187500000\t0.000854492187500000\t0.000854492187500000\t0.000915527343750000\t0.000915527343750000\t0.000915527343750000\t0.000976562500000000\t0.000976562500000000\t0.00103759765625000\t0.00103759765625000\t0.00103759765625000\t0.00109863281250000\t0.00109863281250000\t0.00115966796875000\t0.00115966796875000\t0.00115966796875000\t0.00122070312500000\t0.00122070312500000\t0.00128173828125000\t0.00128173828125000\t0.00134277343750000\t0.00134277343750000\t0.00140380859375000\t0.00140380859375000\t0.00140380859375000\t0.00146484375000000\t0.00146484375000000\t0.00152587890625000\t0.00152587890625000\t0.00158691406250000\t0.00158691406250000\t0.00164794921875000\t0.00164794921875000\t0.00170898437500000\t0.00170898437500000\t0.00177001953125000\t0.00177001953125000\t0.00183105468750000\t0.00183105468750000\t0.00189208984375000\t0.00195312500000000\t0.00195312500000000\t0.00201416015625000\t0.00201416015625000\t0.00207519531250000\t0.00207519531250000\t0.00213623046875000\t0.00213623046875000\t0.00219726562500000\t0.00225830078125000\t0.00225830078125000\t0.00231933593750000\t0.00231933593750000\t0.00238037109375000\t0.00238037109375000\t0.00244140625000000\t0.00250244140625000\t0.00250244140625000\t0.00256347656250000\t0.00256347656250000\t0.00262451171875000\t0.00268554687500000\t0.00268554687500000\t0.00274658203125000\t0.00274658203125000\t0.00280761718750000\t0.00286865234375000\t0.00286865234375000\t0.00292968750000000\t0.00292968750000000\t0.00299072265625000\t0.00305175781250000\t0.00305175781250000\t0.00311279296875000\t0.00311279296875000\t0.00317382812500000\t0.00323486328125000\t0.00323486328125000\t0.00329589843750000\t0.00329589843750000\t0.00335693359375000\t0.00341796875000000\t0.00341796875000000\t0.00347900390625000\t0.00347900390625000\t0.00354003906250000\t0.00360107421875000\t0.00360107421875000\t0.00366210937500000\t0.00366210937500000\t0.00372314453125000\t0.00372314453125000\t0.00378417968750000\t0.00384521484375000\t0.00384521484375000\t0.00390625000000000\t0.00390625000000000\t0.00396728515625000\t0.00396728515625000\t0.00402832031250000\t0.00408935546875000\t0.00408935546875000\t0.00415039062500000\t0.00415039062500000\t0.00421142578125000\t0.00421142578125000\t0.00427246093750000\t0.00427246093750000\t0.00433349609375000\t0.00433349609375000\t0.00439453125000000\t0.00439453125000000\t0.00445556640625000\t0.00445556640625000\t0.00451660156250000\t0.00451660156250000\t0.00457763671875000\t0.00457763671875000\t0.00463867187500000\t0.00463867187500000\t0.00463867187500000\t0.00469970703125000\t0.00469970703125000\t0.00476074218750000\t0.00476074218750000\t0.00482177734375000\t0.00482177734375000\t0.00482177734375000\t0.00488281250000000\t0.00488281250000000\t0.00488281250000000\t0.00494384765625000\t0.00494384765625000\t0.00500488281250000\t0.00500488281250000\t0.00500488281250000\t0.00500488281250000\t0.00506591796875000\t0.00506591796875000\t0.00506591796875000\t0.00512695312500000\t0.00512695312500000\t0.00512695312500000\t0.00512695312500000\t0.00518798828125000\t0.00518798828125000\t0.00518798828125000\t0.00518798828125000\t0.00524902343750000\t0.00524902343750000\t0.00524902343750000\t0.00524902343750000\t0.00524902343750000\t0.00524902343750000\t0.00531005859375000\t0.00531005859375000\t0.00531005859375000\t0.00531005859375000\t0.00531005859375000\t0.00531005859375000\t0.00531005859375000\t0.00531005859375000\t0.00531005859375000\t0.00531005859375000\t0.00537109375000000\t0.00537109375000000\t0.00537109375000000\t0.00537109375000000\t0.00537109375000000\t0.00537109375000000\t0.00537109375000000\t0.00537109375000000\t0.00537109375000000\t0.00531005859375000\t0.00531005859375000\t0.00531005859375000\t0.00531005859375000\t0.00531005859375000\t0.00531005859375000\t0.00531005859375000\t0.00531005859375000\t0.00531005859375000\t0.00531005859375000\t0.00524902343750000\t0.00524902343750000\t0.00524902343750000\t0.00524902343750000\t0.00524902343750000\t0.00524902343750000\t0.00518798828125000\t0.00518798828125000\t0.00518798828125000\t0.00518798828125000\t0.00512695312500000\t0.00512695312500000\t0.00512695312500000\t0.00512695312500000\t0.00506591796875000\t0.00506591796875000\t0.00506591796875000\t0.00500488281250000\t0.00500488281250000\t0.00500488281250000\t0.00500488281250000\t0.00494384765625000\t0.00494384765625000\t0.00488281250000000\t0.00488281250000000\t0.00488281250000000\t0.00482177734375000\t0.00482177734375000\t0.00482177734375000\t0.00476074218750000\t0.00476074218750000\t0.00469970703125000\t0.00469970703125000\t0.00463867187500000\t0.00463867187500000\t0.00463867187500000\t0.00457763671875000\t0.00457763671875000\t0.00451660156250000\t0.00451660156250000\t0.00445556640625000\t0.00445556640625000\t0.00439453125000000\t0.00439453125000000\t0.00433349609375000\t0.00433349609375000\t0.00427246093750000\t0.00427246093750000\t0.00421142578125000\t0.00421142578125000\t0.00415039062500000\t0.00415039062500000\t0.00408935546875000\t0.00408935546875000\t0.00402832031250000\t0.00396728515625000\t0.00396728515625000\t0.00390625000000000\t0.00390625000000000\t0.00384521484375000\t0.00384521484375000\t0.00378417968750000\t0.00372314453125000\t0.00372314453125000\t0.00366210937500000\t0.00366210937500000\t0.00360107421875000\t0.00360107421875000\t0.00354003906250000\t0.00347900390625000\t0.00347900390625000\t0.00341796875000000\t0.00341796875000000\t0.00335693359375000\t0.00329589843750000\t0.00329589843750000\t0.00323486328125000\t0.00323486328125000\t0.00317382812500000\t0.00311279296875000\t0.00311279296875000\t0.00305175781250000\t0.00305175781250000\t0.00299072265625000\t0.00292968750000000\t0.00292968750000000\t0.00286865234375000\t0.00286865234375000\t0.00280761718750000\t0.00274658203125000\t0.00274658203125000\t0.00268554687500000\t0.00268554687500000\t0.00262451171875000\t0.00256347656250000\t0.00256347656250000\t0.00250244140625000\t0.00250244140625000\t0.00244140625000000\t0.00238037109375000\t0.00238037109375000\t0.00231933593750000\t0.00231933593750000\t0.00225830078125000\t0.00225830078125000\t0.00219726562500000\t0.00213623046875000\t0.00213623046875000\t0.00207519531250000\t0.00207519531250000\t0.00201416015625000\t0.00201416015625000\t0.00195312500000000\t0.00195312500000000\t0.00189208984375000\t0.00183105468750000\t0.00183105468750000\t0.00177001953125000\t0.00177001953125000\t0.00170898437500000\t0.00170898437500000\t0.00164794921875000\t0.00164794921875000\t0.00158691406250000\t0.00158691406250000\t0.00152587890625000\t0.00152587890625000\t0.00146484375000000\t0.00146484375000000\t0.00140380859375000\t0.00140380859375000\t0.00140380859375000\t0.00134277343750000\t0.00134277343750000\t0.00128173828125000\t0.00128173828125000\t0.00122070312500000\t0.00122070312500000\t0.00115966796875000\t0.00115966796875000\t0.00115966796875000\t0.00109863281250000\t0.00109863281250000\t0.00103759765625000\t0.00103759765625000\t0.00103759765625000\t0.000976562500000000\t0.000976562500000000\t0.000915527343750000\t0.000915527343750000\t0.000915527343750000\t0.000854492187500000\t0.000854492187500000\t0.000854492187500000\t0.000793457031250000\t0.000793457031250000\t0.000793457031250000\t0.000732421875000000\t0.000732421875000000\t0.000732421875000000\t0.000671386718750000\t0.000671386718750000\t0.000671386718750000\t0.000610351562500000\t0.000610351562500000\t0.000610351562500000\t0.000610351562500000\t0.000549316406250000\t0.000549316406250000\t0.000549316406250000\t0.000488281250000000\t0.000488281250000000\t0.000488281250000000\t0.000488281250000000\t0.000427246093750000\t0.000427246093750000\t0.000427246093750000\t0.000427246093750000\t0.000427246093750000\t0.000366210937500000\t0.000366210937500000\t0.000366210937500000\t0.000366210937500000\t0.000366210937500000\t0.000305175781250000\t0.000305175781250000\t0.000305175781250000\t0.000305175781250000\t0.000305175781250000\t0.000244140625000000\t0.000244140625000000\t0.000244140625000000\t0.000244140625000000\t0.000244140625000000\t0.000244140625000000\t0.000183105468750000\t0.000183105468750000\t0.000183105468750000\t0.000183105468750000\t0.000183105468750000\t0.000183105468750000\t0.000183105468750000\t0.000183105468750000\t0.000122070312500000\t0.000122070312500000\t0.000122070312500000\t0.000122070312500000\t0.000122070312500000\t0.000122070312500000\t0.000122070312500000\t0.000122070312500000\t0.000122070312500000\t6.10351562500000e-05\t6.10351562500000e-05\t6.10351562500000e-05\t6.10351562500000e-05\t6.10351562500000e-05\t6.10351562500000e-05\t6.10351562500000e-05\t6.10351562500000e-05\t6.10351562500000e-05\t6.10351562500000e-05\t6.10351562500000e-05\t6.10351562500000e-05\t6.10351562500000e-05\t6.10351562500000e-05\t0\t0\t0\t0\t0\t0\t0\t0\t0\t0\t0\t0\t0\t0\t0\t0\t0\t0\t0\t0\t0\t0\t0\t0\t0\t0\t0\t0\t0\t0\t0\t0\t0\t0\t0\t0\t0\t0\t0\t0\t0\t0\t0\t0\t0\t0\t0\t0\t0\t0\t0\t0\t0\t0\t0\t0\t0\t0\t0\t0\t0\t0\t0\t0\t0\t0\t0\t0\t0\t0\t0\t0\t0\t0\t0\t0\t0\t0\t0\t0\t0\t0\t0\t0\t0\t0\t0\t0\t0\t0\t0\t0\t0\t0\t0\t0\t0\t0\t0\t0\t0\t0\t0\t0\t0\t0\t0\t0\t0\t0\t0]"
  Rate Transition4 : RateTransition  Commented=on
  SpectrumMeasure : Subsystem  Commented=on
  Subsystem : Subsystem
  Subsystem1 : Subsystem
  Subsystem2 : Subsystem
  Subsystem3 : Subsystem
  Subsystem4 : Subsystem
  Subsystem5 : Subsystem
  Subsystem6 : Subsystem
  Subsystem7 : Subsystem
  Sum : Sum  Inputs=|++++++++
  Triggered Subsystem : Subsystem  Commented=on  TreatAsAtomicUnit=on
  Unit Delay{1..7} (7 alike) : UnitDelay  SampleTime=-1  HasFrameUpgradeWarning=on
  u : Outport
  wires:
  Unit Delay1/1 -> Subsystem1/1(In1), Unit Delay2/1
  Unit Delay5/1 -> Subsystem5/1(In1), Unit Delay6/1
  In1/1 -> Subsystem/1(In1), Unit Delay1/1
  Unit Delay2/1 -> Subsystem2/1(In1), Unit Delay3/1
  Unit Delay3/1 -> Unit Delay4/1, Subsystem3/1(In1)
  Unit Delay4/1 -> Subsystem4/1(In1), Unit Delay5/1
  Unit Delay6/1 -> Subsystem6/1(In1), Unit Delay7/1
  Unit Delay7/1 -> Subsystem7/1(In1)
  Subsystem/1(Out1) -> Sum/1
  Subsystem1/1(Out1) -> Sum/2
  Subsystem2/1(Out1) -> Sum/3
  Subsystem3/1(Out1) -> Sum/4
  Subsystem4/1(Out1) -> Sum/5
  Subsystem5/1(Out1) -> Sum/6
  Subsystem6/1(Out1) -> Sum/7
  Subsystem7/1(Out1) -> Sum/8
  Sum/1 -> Compare To Constant/1
  Compare To Constant/1 -> u/1

== system Simple_Model_Packaging_4_1/接收端本地载波 ==
  note: 此处无延时
  note: 该条支路对接收端的本地载波进行建模，从而建模相干解调过程
  note: 此处延时5e-6
  In1 : Inport
  Buffer9 : Buffer  N=model.parameter.Buffer9.Output_buffer_size  OutputFrames=off
  Conj : Math  Operator=conj
  Delay5 : dspobslib/Delay  InputProcessing=Columns as channels (frame based)  dly_unit=Samples  delay=model.parameter.Delay5.samples_length  ic_detail=off  dif_ic_for_ch=on  dif_ic_for_dly=off  ic=0  reset_popup=None
  Out1 : Outport
  wires:
  Conj/1 -> Buffer9/1
  In1/1 -> Conj/1
  Buffer9/1 -> Delay5/1
  Delay5/1 -> Out1/1

== system Simple_Model_Packaging_4_1/本地载波生成模块 ==
  note: 帧信号对应的本地载波生成
  Constant : Constant  Value=model.parameter.Func1.f_chirp_min
  Constant1 : Constant  Value=model.parameter.Func1.f_chirp_max
  Constant2 : Constant  Value=model.parameter.Func1.T_chirp
  Digital Clock1 : DigitalClock  SampleTime=model.parameter.Digital_Clock2.CarrierTs
  MATLAB Function : MATLAB Function  TreatAsAtomicUnit=on
  Carrier : Outport
  wires:
  Digital Clock1/1 -> MATLAB Function/1(t)
  MATLAB Function/1(y) -> Carrier/1  "本地载波"
  Constant/1 -> MATLAB Function/2(f_chirp_min)
  Constant1/1 -> MATLAB Function/3(f_chirp_max)
  Constant2/1 -> MATLAB Function/4(T_chirp)

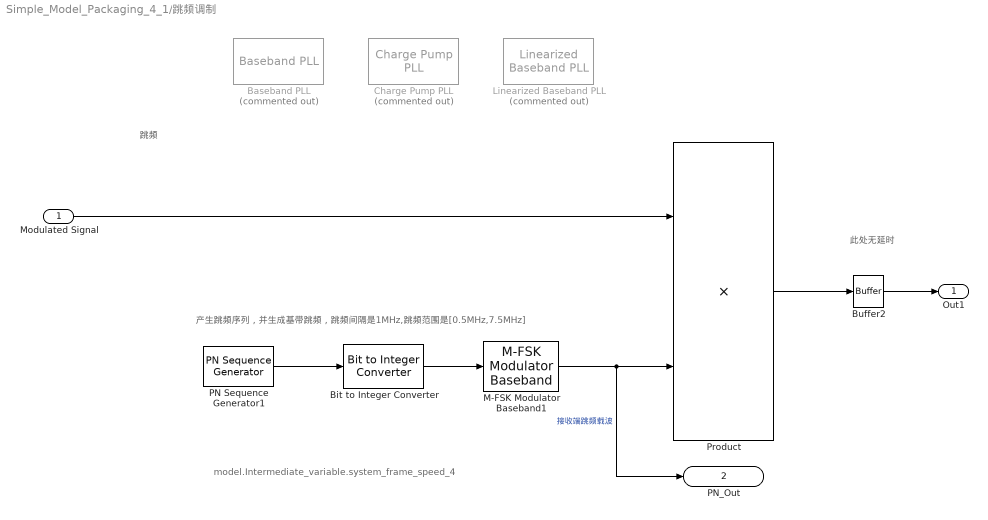
== system Simple_Model_Packaging_4_1/跳频调制 ==
  note: model.Intermediate_variable.system_frame_speed_4
  note: 跳频
  note: 此处无延时
  note: 产生跳频序列，并生成基带跳频，跳频间隔是1MHz,跳频范围是[0.5MHz,7.5MHz]
  Modulated Signal : Inport
  Baseband PLL : commsynccomp2/Baseband PLL  Commented=on  Fn="[3.0002  0  40002]"  Fd="[1   67.46   2270.9   40002]"  Kvco=1
  Bit to Integer Converter : simulink/Logic and Bit Operations/Bit to Integer Converter  nbits=model.parameter.Bit_to_Integer_Converter.M  bitOrder=MSB first  signedOutputValues=Unsigned  outDtype=double  outDtypeSigned=Inherit via internal rule
  Buffer2 : Buffer  N=model.parameter.Buffer2.Output_buffer_size  OutputFrames=off
  Charge Pump PLL : commsynccomp2/Charge Pump PLL  Commented=on  Fn="[3.0002  0  40002]"  Fd="[1   67.46   2270.9   40002]"  Kvco=1  Fc=100  Ph=0  Ac=1
  Linearized Baseband PLL : commsynccomp2/Linearized Baseband PLL  Commented=on  Fn="[3.0002  0  40002]"  Fd="[1   67.46   2270.9   40002]"  Kvco=1
  M-FSK Modulator Baseband1 : commdigbbndfm2/M-FSK Modulator Baseband  M=model.parameter.M_FSK_Modulator_Baseband1.M_ary_number  InType=Integer  Enc=Gray  freqSep=model.parameter.M_FSK_Modulator_Baseband1.Frequency_separation  phaseType=Continuous  numSamp=model.parameter.M_FSK_Modulator_Baseband1.Samples_per_symbol  RateOptions=Enforce single-rate processing  outDataType=double
  PN Sequence Generator1 : commseqgen3/PN Sequence Generator  poly=model.parameter.PN_Sequence_Generator1.Generator_polynomial  ini_sta=model.parameter.PN_Sequence_Generator1.Initial_states  outBitMaskSource=Dialog parameter  shift=0  outVarSiz=off  maxOutSizeMode=Dialog parameter  maxOutSize=[10 1]  Ts=model.parameter.PN_Sequence_Generator1.Sample_time  sampPerFrame=model.parameter.PN_Sequence_Generator1.Samples_per_frame  reset=off  bitPackedOutputs=off  outDataType=double  numPackedBits=5  bitPackDataSigned=off  bitPackedOutDType=double
  Product : Product
  Out1 : Outport
  PN_Out : Outport  Port=2
  wires:
  M-FSK Modulator Baseband1/1 -> PN_Out/1, Product/2  "接收端跳频载波"
  Product/1 -> Buffer2/1
  Buffer2/1 -> Out1/1
  Modulated Signal/1 -> Product/1
  PN Sequence Generator1/1 -> Bit to Integer Converter/1
  Bit to Integer Converter/1 -> M-FSK Modulator Baseband1/1

== system Simple_Model_Packaging_4_1/间歇PN码与接收端信源的时序同步 ==
  note: 对RS解码后的信号和接收端对应的间歇PN码截取正确码元部分，去除由于延时导致的
      | 不正确RS解码bit
  In1 : Inport
  In2 : Inport  Port=2
  发送端的间歇PN码 : Product
  Out1 : Outport
  wires:
  In2/1 -> 发送端的间歇PN码/2
  发送端的间歇PN码/1 -> Out1/1
  In1/1 -> 发送端的间歇PN码/1

== system Simple_Model_Packaging_4_1/信源RS解码/If Action Subsystem1 ==
  In1 : Inport
  Action Port : ActionPort  ActionPortLabel=if(u1 == 1)
  Out1 : Outport
  wires:
  In1/1 -> Out1/1

== system Simple_Model_Packaging_4_1/信源RS解码/If Action Subsystem4 ==
  In1 : Inport
  Action Port : ActionPort  ActionPortLabel=else
  Out1 : Outport
  wires:
  In1/1 -> Out1/1

== system Simple_Model_Packaging_4_1/信源基带解调/Baseband Signal Selector Rx ==
  In1 : Inport
  Constant : Constant  Value=model.user_defined.TR.Baseband_Modulation_type
  If : If  IfExpression=u1 == 1  ElseIfExpressions=u1 == 2
  If Action Subsystem1 : Subsystem  TreatAsAtomicUnit=on
  If Action Subsystem4 : Subsystem  TreatAsAtomicUnit=on
  If Action Subsystem5 : Subsystem  TreatAsAtomicUnit=on
  Merge : Merge  Inputs=3
  Out1 : Outport
  wires:
  In1/1 -> If Action Subsystem4/1(In1), If Action Subsystem1/1(In1), If Action Subsystem5/1(In1)
  If Action Subsystem5/1(Out1) -> Merge/3
  If Action Subsystem1/1(Out1) -> Merge/2
  If Action Subsystem4/1(Out1) -> Merge/1
  Constant/1 -> If/1
  Merge/1 -> Out1/1
  If/3 -> If Action Subsystem5/Action
  If/1 -> If Action Subsystem4/Action
  If/2 -> If Action Subsystem1/Action

== system Simple_Model_Packaging_4_1/信源部分基带调制/Baseband Signal Selector Tx ==
  In1 : Inport
  Constant : Constant  Value=model.user_defined.TR.Baseband_Modulation_type
  If : If  IfExpression=u1 == 1  ElseIfExpressions=u1 == 2
  If Action Subsystem1 : Subsystem  TreatAsAtomicUnit=on
  If Action Subsystem4 : Subsystem  TreatAsAtomicUnit=on
  If Action Subsystem5 : Subsystem  TreatAsAtomicUnit=on
  Merge : Merge  Inputs=3
  Out1 : Outport
  wires:
  If Action Subsystem5/1(Out1) -> Merge/3
  Constant/1 -> If/1
  Merge/1 -> Out1/1
  If/3 -> If Action Subsystem5/Action
  If/1 -> If Action Subsystem4/Action
  If/2 -> If Action Subsystem1/Action
  If Action Subsystem1/1(Out1) -> Merge/2
  If Action Subsystem4/1(Out1) -> Merge/1
  In1/1 -> If Action Subsystem4/1(In1), If Action Subsystem1/1(In1), If Action Subsystem5/1(In1)

== system Simple_Model_Packaging_4_1/信源部分基带调制/If Action Subsystem1 ==
  In1 : Inport
  Action Port : ActionPort  ActionPortLabel=else
  Out1 : Outport
  wires:
  In1/1 -> Out1/1

== system Simple_Model_Packaging_4_1/信源部分基带调制/If Action Subsystem4 ==
  In1 : Inport
  Action Port : ActionPort  ActionPortLabel=if(u1 == 1)
  Out1 : Outport
  wires:
  In1/1 -> Out1/1

== system Simple_Model_Packaging_4_1/帧信号和信源信号混合/Subsystem ==
  In1 : Inport
  AWGN Channel : commchan3/AWGN Channel  InputProcessing=Columns as channels (frame based)  seed=67  noiseMode="Signal to noise ratio  (SNR)"  EbNodB=10  EsNodB=10  SNRdB=model.parameter.Awgn.SNR  bitsPerSym=1  Ps=model.parameter.Awgn.input_power  Tsym=1  variance=1
  Add : Sum
  NosieGen : Subsystem
  Out1 : Outport
  wires:
  In1/1 -> Add/2
  AWGN Channel/1 -> Out1/1
  NosieGen/1(Jamming_Signal_Output) -> Add/1  "TRSignal"
  Add/1 -> AWGN Channel/1

== system Simple_Model_Packaging_4_1/帧序列识别器/SpectrumMeasure ==
  y : Inport
  Buffer5 : Buffer  N=1  OutputFrames=off
  Rate Transition1 : RateTransition  Commented=on  OutPortSampleTime=1e-8
  Spectrum Analyzer2 : SpectrumAnalyzer
  wires:
  y/1 -> Buffer5/1
  Buffer5/1 -> Spectrum Analyzer2/1

== system Simple_Model_Packaging_4_1/帧序列识别器/Subsystem ==
  In1 : Inport
  Constant : Constant
  Constant1 : Constant  Value=-1
  If : If  IfExpression=u1 ==0
  If Action Subsystem : Subsystem  TreatAsAtomicUnit=on
  If Action Subsystem1 : Subsystem  TreatAsAtomicUnit=on
  Merge : Merge
  Out1 : Outport
  wires:
  Constant/1 -> If Action Subsystem/1(In1)
  Constant1/1 -> If Action Subsystem1/1(In1)
  Merge/1 -> Out1/1
  If/1 -> If Action Subsystem/Action
  If Action Subsystem/1(Out1) -> Merge/1
  In1/1 -> If/1
  If/2 -> If Action Subsystem1/Action
  If Action Subsystem1/1(Out1) -> Merge/2

== system Simple_Model_Packaging_4_1/帧序列识别器/Subsystem1 ==
  In1 : Inport
  Constant : Constant
  Constant1 : Constant  Value=-1
  If : If  IfExpression=u1 ==3
  If Action Subsystem : Subsystem  TreatAsAtomicUnit=on
  If Action Subsystem1 : Subsystem  TreatAsAtomicUnit=on
  Merge : Merge
  Out1 : Outport
  wires:
  Constant/1 -> If Action Subsystem/1(In1)
  Constant1/1 -> If Action Subsystem1/1(In1)
  Merge/1 -> Out1/1
  If/1 -> If Action Subsystem/Action
  If Action Subsystem/1(Out1) -> Merge/1
  In1/1 -> If/1
  If/2 -> If Action Subsystem1/Action
  If Action Subsystem1/1(Out1) -> Merge/2
